simulink model "encoder_read_test"  (R2019a)
settings: Solver=FixedStepAuto  StartTime=0.0  StopTime=inf  RelTol=1e-3  EnableMultiTasking=on
libraries: raspberrypilib x2
settings Model: SimulationMode=external  Creator=mnimi  LastModifiedBy=emiel
settings SolverCC: PositivePriorityOrder=on
settings DataIOCC: ReturnWorkspaceOutputs=off
settings OptimizationCC: EnhancedBackFolding=on  PassReuseOutputArgsAs=Individual arguments  MaxStackSize=64  OptimizeBlockOrder=speed  DifferentSizesBufferReuse=on  OptimizationCustomize=off
settings DebuggingCC: ParameterTunabilityLossMsg=error  ArithmeticOperatorsInVariantConditions=warning
settings HardwareCC: ProdBitPerPointer=32  ProdBitPerSizeT=32  ProdBitPerPtrDiffT=32  ProdLargestAtomicInteger=Long  ProdLargestAtomicFloat=Double  ProdEndianess=BigEndian  ProdWordSize=32  ProdHWDeviceType=ARM Compatible->ARM Cortex
settings ModelReferenceCC: UpdateModelReferenceTargets=Force
settings SFSimCC: MATLABDynamicMemAlloc=off
settings RTWCC: SystemTargetFile=ert.tlc  HardwareBoard=Raspberry Pi  TLCOptions="-aInlineSetEventsForThisBaseRateFcn=TLC_FALSE -aSuppressMultiTaskScheduler=TLC_FALSE  -aRateBasedStepFcn=0"  TemplateMakefile=ert_default_tmf  Toolchain=GNU GCC Raspberry Pi  BuildConfiguration=Faster Runs  IncludeHyperlinkInReport=on
settings CodeAppCC: ForceParamTrailComments=on  IgnoreCustomStorageClasses=off  OperatorAnnotations=on  SimulinkDataObjDesc=on  SFDataObjDesc=on  InsertBlockDesc=on
settings ERTTargetCC: SupportContinuousTime=on  SupportVariableSizeSignals=on

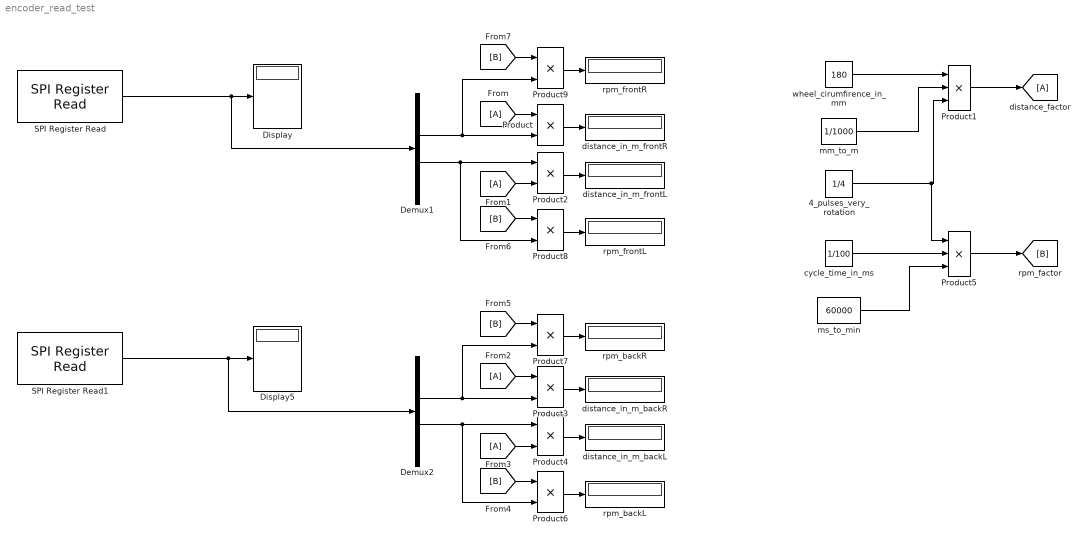
== system encoder_read_test ==
  4_pulses_very_rotation : Constant  Value=1/4
  Demux1 : Demux
  Demux2 : Demux
  Display : Display
  Display5 : Display
  Product{,2..4,6..9} (8 alike) : Product
  Product1 : Product  Inputs=3
  Product5 : Product  Inputs=3
  SPI Register Read : raspberrypilib/SPI Register Read  BoardProperty=Pi 3 Model B+  SPIModule=uint32(0)  Mode=Master  BusSpeed=1000000  Pin=SPI0_CE0  FirstBitToTransfer=Most significant bit (MSB)  ClockMode=0  BlockFunction=Read  RegisterAddress=0  OutputDataType=uint8  OutputDataLength=4  SampleTime=0.1
      settings: SourceProductName=Simulink Support Package for Raspberry Pi Hardware  SourceProductBaseCode=RASPPI
  SPI Register Read1 : raspberrypilib/SPI Register Read  BoardProperty=Pi 3 Model B+  SPIModule=uint32(0)  Mode=Master  BusSpeed=1000000  Pin=SPI0_CE1  FirstBitToTransfer=Most significant bit (MSB)  ClockMode=0  BlockFunction=Read  RegisterAddress=0  OutputDataType=uint8  OutputDataLength=4  SampleTime=0.1
      settings: SourceProductName=Simulink Support Package for Raspberry Pi Hardware  SourceProductBaseCode=RASPPI
  cycle_time_in_ms : Constant  Value=1/100
  distance_in_m_backL : Display
  distance_in_m_backR : Display
  distance_in_m_frontL : Display
  distance_in_m_frontR : Display
  mm_to_m : Constant  Value=1/1000
  ms_to_min : Constant  Value=60000
  rpm_backL : Display
  rpm_backR : Display
  rpm_frontL : Display
  rpm_frontR : Display
  wheel_cirumfirence_in_mm : Constant  Value=180
  wires:
  SPI Register Read/1 -> Display/1, Demux1/1
  SPI Register Read1/1 -> Display5/1, Demux2/1
  wheel_cirumfirence_in_mm/1 -> Product1/1
  mm_to_m/1 -> Product1/2
  Product1/1 -> [A]
  4_pulses_very_rotation/1 -> Product5/1, Product1/3
  [A] -> Product/1
  Demux1/2 -> Product9/2, Product/2
  Product/1 -> distance_in_m_frontR/1
  Demux1/3 -> Product8/2, Product2/1
  [A] -> Product2/2
  Product2/1 -> distance_in_m_frontL/1
  Demux2/2 -> Product7/2, Product3/2
  [A] -> Product3/1
  Demux2/3 -> Product6/2, Product4/1
  Product3/1 -> distance_in_m_backR/1
  Product4/1 -> distance_in_m_backL/1
  [A] -> Product4/2
  cycle_time_in_ms/1 -> Product5/2
  ms_to_min/1 -> Product5/3
  Product5/1 -> [B]
  [B] -> Product6/1
  Product6/1 -> rpm_backL/1
  Product7/1 -> rpm_backR/1
  [B] -> Product7/1
  Product8/1 -> rpm_frontL/1
  [B] -> Product8/1
  Product9/1 -> rpm_frontR/1
  [B] -> Product9/1
